simulink library "lib_controls"  (Simulink 7.9)
settings: Solver=ode45  SolverMode=SingleTasking  StartTime=0.0  StopTime=10.0  RelTol=1e-3
undefined symbols (not defined in the file): amb_tmp, cs_charge_deplete_bool, cs_charge_pwr, cs_charge_trq, cs_clt_tmp, cs_decel_fc_off, cs_decel_regen_threshold, cs_dl_assist_trq_threshold, cs_dl_regen_trq_threshold, cs_electric_decel_spd, cs_electric_launch_spd, cs_electric_launch_spd_hi, cs_electric_launch_spd_lo, cs_eng_min_spd, cs_eng_on_soc, cs_fc_init_state, cs_fc_max_pwr_frac, cs_fc_min_pwr_frac, cs_fc_on, cs_fc_pwr_opt, cs_fc_spd_opt, cs_fuzzy_fuel_mode, cs_hi_soc, cs_hi_trq_frac, cs_lo_soc, cs_lo_trq_frac, cs_max_gc_spd, cs_max_pwr, cs_max_pwr_fall_rate, cs_max_pwr_rise_rate, cs_mc_assist_max_frac, cs_mc_assist_min_frac, cs_mc_assist_slope, cs_mc_regen_max_frac, cs_mc_regen_min_frac, cs_mc_regen_slope, cs_mean_eff, cs_mean_eff_bool, cs_min_gc_spd, cs_min_off_time, cs_min_pwr, cs_min_trq_frac, cs_mph_avg_time, cs_off_trq_frac, cs_plot_output, cs_pwr, cs_regen_avg_time, cs_scale_factor, cs_shutoff, cs_soc_range, cs_spd, cs_target_soc, cs_trq_to_soc_factor, cvt_locus_pwr, cvt_locus_spd, cyc_mph, enable_sim_stop_distance, enable_sim_stop_max_spd, enable_sim_stop_speed, enable_sim_stop_time ... (+110)
libraries: lib_controls x124, simulink3 x18, lib_etc x1
(part 13 of 17)

== system lib_controls/<vc> par auto s/a/gearbox control for use w/ AT  in parallel sa/downshift  command1 ==
  prev gear number : Inport
  engine load : Inport  Port=2
  engine speed : Inport  Port=3
  Mux : Mux  Inputs=2
  Relational Operator : RelationalOperator  Operator=>  InputSameDT=on
  load fraction : Subsystem  mask(Gear Selector){spd=gb_dnshift_spd, load=gb_dnshift_load}
      mask prompts: spd "Speeds:"; load "Load Fractions:"
      mask help:
      | This block will perform a linear interplation (extrapolation outside of bounds) to determine the shift point load fraction associated with the current gear number and speed.
      |
      | The Speeds parameter should be defined as an array of vectors containing speeds for each gear number.  The Load Fractions parameter should be defined as a array of vectors containing load fractions indexed by the speeds in the Speeds parameter for each gear number.
      mask Help:
      | Reference the base workspace variables - gb_**shift_spd and gb_**shift_load  where ** is either up for upshift conditions or dn for downshift conditions.
      | 
      | Or define the arrays as follows:
      | 
      | {[spd1 spd2 spd3 spd4]; [spd1 spd2 spd3 spd4]; ...}
      | 
      | {[load1 load2 load3 load4]; [load1 load2 load3 load4]; ...}
      | 
      | where each array contains one row for each gear in the gearbox.  Speeds should be defined in rad/s and loads as a decimal fraction.
  command : Outport  InitialOutput=0
  wires:
  engine speed/1 -> Mux/2
  load fraction/1(Out1) -> Relational Operator/2
  Mux/1 -> load fraction/1(In1)
  engine load/1 -> Relational Operator/1
  prev gear number/1 -> Mux/1
  Relational Operator/1 -> command/1

== system lib_controls/<vc> par auto s/a/gearbox control for use w/ AT  in parallel sa/est. engine trq and spd ==
  prev gear number : Inport
  " prev eta_gb" : Inport  Port=2
  gb_trq_out_r : Inport  Port=3
  gb_spd_out_r : Inport  Port=4
  Block NOTES : Subsystem
      mask Display: disp('Block\nNOTES')
  Constant2 : Constant  Value=[1 1]
  Constant5 : Constant  Value=0
  Demux : Demux  Outputs=2
  K_adv : Subsystem
  Logical Operator : Logic
  Logical Operator1 : Logic  Operator=NOT  Inputs=1
  Memory : Memory
  Mux1 : Mux  Inputs=2
  Mux2 : Mux  Inputs=2
  Relational Operator1 : RelationalOperator  Operator=>  InputSameDT=on
  SR Look-Up Table SR=wout/win : Lookup  InputValues=htc_k_adv  Table=htc_sr  SaturateOnIntegerOverflow=on
  Saturation1 : Saturate  UpperLimit=1  LowerLimit=0.7
  Saturation2 : Saturate  UpperLimit=inf  LowerLimit=0
  Switch : Switch  Threshold=eps  SaturateOnIntegerOverflow=on  InputSameDT=on
  TR Look-Up Table TR=Tout/Tin : Lookup  InputValues=htc_k_adv  Table=htc_tr  SaturateOnIntegerOverflow=on
  TR,SR : Mux  Inputs=2
  gear ratio1 : Lookup  InputValues=[1:length(gb_ratio)]  Table=gb_ratio  SaturateOnIntegerOverflow=on
  ~eng trq and spd : Product  Inputs=*/  SaturateOnIntegerOverflow=on  RndMeth=Zero  InputSameDT=on  OutDataTypeStr=Inherit: Same as first input
  ~gb_spd_in_r : Product  SaturateOnIntegerOverflow=on  RndMeth=Zero  InputSameDT=on  OutDataTypeStr=Inherit: Same as first input
  ~gb_trq_in_r : Product  Inputs=//*  SaturateOnIntegerOverflow=on  RndMeth=Zero  InputSameDT=on  OutDataTypeStr=Inherit: Same as first input
  est eng trq (Nm) : Outport
  est eng spd (rad/s) : Outport  Port=2
  gb_spd_in_est (rad/s)1 : Outport  Port=3
  wires:
  ~gb_spd_in_r/1 -> Mux2/2, gb_spd_in_est (rad/s)1/1, Mux1/2
  ~gb_trq_in_r/1 -> Relational Operator1/1, Mux1/1, Mux2/1
  SR Look-Up Table SR=wout/win/1 -> TR,SR/2
  TR Look-Up Table TR=Tout/Tin/1 -> TR,SR/1
  K_adv/1(K_adv) -> SR Look-Up Table SR=wout/win/1, TR Look-Up Table TR=Tout/Tin/1
  Mux2/1 -> K_adv/1("Req'd output trq and spd (Nm), (rad/s)")
  ~eng trq and spd/1 -> Demux/1
  Mux1/1 -> ~eng trq and spd/1
  [locked_up] -> Memory/1
  Logical Operator/1 -> Switch/2
  Logical Operator1/1 -> Logical Operator/2
  Memory/1 -> Logical Operator1/1
  Demux/1 -> est eng trq (Nm)/1
  prev gear number/1 -> gear ratio1/1
  Relational Operator1/1 -> Logical Operator/1
  Constant5/1 -> Relational Operator1/2
  Saturation2/1 -> est eng spd (rad/s)/1
  Demux/2 -> Saturation2/1
  Saturation1/1 -> ~gb_trq_in_r/2
  " prev eta_gb"/1 -> Saturation1/1
  Switch/1 -> ~eng trq and spd/2
  Constant2/1 -> Switch/3
  TR,SR/1 -> Switch/1
  gear ratio1/1 -> ~gb_spd_in_r/1, ~gb_trq_in_r/1
  gb_spd_out_r/1 -> ~gb_spd_in_r/2
  gb_trq_out_r/1 -> ~gb_trq_in_r/3

== system lib_controls/<vc> par auto s/a/gearbox control for use w/ AT  in parallel sa/est. engine trq and spd assuming lockup ==
  new gear number : Inport
  " prev eta_gb" : Inport  Port=2
  gb_trq_out_r : Inport  Port=3
  gb_spd_in_est : Inport  Port=4
  Block NOTES : Subsystem
      mask Display: disp('Block\nNOTES')
  Memory : Memory  X0=gb_ratio(1)
  Saturation1 : Saturate  UpperLimit=1  LowerLimit=0.7
  Saturation2 : Saturate  UpperLimit=inf  LowerLimit=0
  gear ratio1 : Lookup  InputValues=[1:length(gb_ratio)]  Table=gb_ratio  SaturateOnIntegerOverflow=on
  ~gb_spd_in_r : Product  Inputs=*/*  SaturateOnIntegerOverflow=on  RndMeth=Zero  InputSameDT=on  OutDataTypeStr=Inherit: Same as first input
  ~gb_trq_in_r : Product  Inputs=//*  SaturateOnIntegerOverflow=on  RndMeth=Zero  InputSameDT=on  OutDataTypeStr=Inherit: Same as first input
  est eng trq (Nm) : Outport
  est eng spd (rad/s) : Outport  Port=2
  wires:
  ~gb_spd_in_r/1 -> Saturation2/1
  ~gb_trq_in_r/1 -> est eng trq (Nm)/1
  gb_spd_in_est/1 -> ~gb_spd_in_r/3
  Memory/1 -> ~gb_spd_in_r/2
  Saturation2/1 -> est eng spd (rad/s)/1
  new gear number/1 -> gear ratio1/1
  gb_trq_out_r/1 -> ~gb_trq_in_r/3
  gear ratio1/1 -> Memory/1, ~gb_spd_in_r/1, ~gb_trq_in_r/1
  " prev eta_gb"/1 -> Saturation1/1
  Saturation1/1 -> ~gb_trq_in_r/2

== system lib_controls/<vc> par auto s/a/gearbox control for use w/ AT  in parallel sa/shifting1 ==
  gear number : Inport
  Constant : Constant  Value=gb_shift_delay-1e-6
  Relational Operator : RelationalOperator  Operator=<  InputSameDT=on
  time since last shift : Subsystem
      mask Display: disp('time since\nlast shift')
  out_1 : Outport  InitialOutput=0
  wires:
  Relational Operator/1 -> out_1/1
  gear number/1 -> time since last shift/1(in_1)
  Constant/1 -> Relational Operator/2
  time since last shift/1(out_1) -> Relational Operator/1

== system lib_controls/<vc> par auto s/a/gearbox control for use w/ AT  in parallel sa/upshift  command ==
  prev gear number : Inport
  engine load : Inport  Port=2
  engine speed : Inport  Port=3
  Mux : Mux  Inputs=2
  Relational Operator : RelationalOperator  Operator=<  InputSameDT=on
  load fraction : Subsystem  mask(Gear Selector){spd=gb_upshift_spd, load=gb_upshift_load}
      mask prompts: spd "Speeds:"; load "Load Fractions:"
      mask help:
      | This block will perform a linear interplation (extrapolation outside of bounds) to determine the shift point load fraction associated with the current gear number and speed.
      |
      | The Speeds parameter should be defined as an array of vectors containing speeds for each gear number.  The Load Fractions parameter should be defined as a array of vectors containing load fractions indexed by the speeds in the Speeds parameter for each gear number.
      mask Help:
      | Reference the base workspace variables - gb_**shift_spd and gb_**shift_load  where ** is either up for upshift conditions or dn for downshift conditions.
      | 
      | Or define the arrays as follows:
      | 
      | {[spd1 spd2 spd3 spd4]; [spd1 spd2 spd3 spd4]; ...}
      | 
      | {[load1 load2 load3 load4]; [load1 load2 load3 load4]; ...}
      | 
      | where each array contains one row for each gear in the gearbox.  Speeds should be defined in rad/s and loads as a decimal fraction.
  command : Outport  InitialOutput=0
  wires:
  Relational Operator/1 -> command/1
  engine speed/1 -> Mux/2
  Mux/1 -> load fraction/1(In1)
  prev gear number/1 -> Mux/1
  engine load/1 -> Relational Operator/1
  load fraction/1(Out1) -> Relational Operator/2

== system lib_controls/<vc> par auto s/a/motor controller logic/Block NOTES ==
  note: This block models a motor/controller's logic, modulating the power input requirement as follows:
      | - enforcing the maximum current limit of the motor/controller
      | - shutting the motor off if the average speed over the time step ==0
      | - shutting the motor off if the transmission is shifting.

== system lib_controls/<vc> par auto s/a/motor controller logic/Sign ==
  in_1 : Inport
  Constant : Constant  Value=0
  Relational Operator : RelationalOperator  Operator=>  InputSameDT=on
  Relational Operator1 : RelationalOperator  Operator=<  InputSameDT=on
  Sum : Sum  Inputs=+-  SaturateOnIntegerOverflow=on  InputSameDT=on  OutDataTypeStr=Inherit: Same as first input
  out_1 : Outport  InitialOutput=0
  wires:
  in_1/1 -> Relational Operator/1, Relational Operator1/1
  Constant/1 -> Relational Operator1/2, Relational Operator/2
  Relational Operator1/1 -> Sum/2
  Relational Operator/1 -> Sum/1
  Sum/1 -> out_1/1

== system lib_controls/<vc> par balanced/engine on (balanced parallel hybrid)/Block NOTES1 ==
  note: Engine is on if,
      | 1) engine was on previously and engine is not warm
      | 2) engine was on and is shifting
      | 3) battery power is insufficient
      | 4) (speed is less than electric launch speed OR soc is less than
      | lo soc unless charge depleting) AND
      | soc is less than hi soc AND
      | trq frac is greater than lo trq frac OR soc is less than mean of hi and
      | lo soc unless charge depleting AND
      | (trq is too high AND speed is too high for idle) OR engine is allowed to idle

== system lib_controls/<vc> par balanced/engine on (balanced parallel hybrid)/Subsystem ==
  in_1 : Inport
  Clock : Clock
  Constant1 : Constant  Value=n
  Constant2 : Constant
  Integrator : Integrator
  Memory : Memory  X0=-0.1
  Memory1 : Memory
  Product : Product  Inputs=*/  SaturateOnIntegerOverflow=on  RndMeth=Zero  InputSameDT=on  OutDataTypeStr=Inherit: Same as first input
  Product1 : Product  SaturateOnIntegerOverflow=on  RndMeth=Zero  InputSameDT=on  OutDataTypeStr=Inherit: Same as first input
  Relational Operator : RelationalOperator  Operator=<=  InputSameDT=on
  Sum : Sum  Inputs=+-  SaturateOnIntegerOverflow=on  InputSameDT=on  OutDataTypeStr=Inherit: Same as first input
  Sum1 : Sum  Inputs=|+-  SaturateOnIntegerOverflow=on  InputSameDT=on  OutDataTypeStr=Inherit: Same as first input
  Switch{,1..3} (4 alike) : Switch  Threshold=eps  SaturateOnIntegerOverflow=on  InputSameDT=on
  Variable Transport Delay : VariableTransportDelay  MaximumDelay=n
  out_1 : Outport  InitialOutput=0
  wires:
  Product/1 -> out_1/1
  Sum/1 -> Product/1
  Variable Transport Delay/1 -> Sum/2
  Integrator/1 -> Variable Transport Delay/1, Sum/1
  Relational Operator/1 -> Switch/2
  Constant1/1 -> Product1/2
  Clock/1 -> Sum1/1, Memory/1, Relational Operator/1, Switch/1
  Memory/1 -> Sum1/2
  Sum1/1 -> Product1/1
  Product1/1 -> Relational Operator/2, Switch/3
  Switch/1 -> Variable Transport Delay/2, Switch1/2, Switch1/1
  Constant2/1 -> Switch1/3
  Switch1/1 -> Product/2
  Switch2/1 -> Integrator/1
  Switch3/1 -> Memory1/1
  in_1/1 -> Switch2/3, Switch3/3
  Memory1/1 -> Switch2/1, Switch3/1
  [shifting] -> Switch2/2, Switch3/2

== system lib_controls/<vc> par balanced/engine on (balanced parallel hybrid)/key_on ==
  Clock : Clock
  Fcn1 : Fcn  Expr=rem(u[1],period)
  Look-Up Table : Lookup  InputValues=t  Table=y  SaturateOnIntegerOverflow=on
  out_1 : Outport  InitialOutput=0
  wires:
  Fcn1/1 -> Look-Up Table/1
  Clock/1 -> Fcn1/1
  Look-Up Table/1 -> out_1/1

== system lib_controls/<vc> par balanced/engine on (balanced parallel hybrid)/repeated cycle:  speed required at end of NEXT step ==
  Clock : Clock
  Fcn1 : Fcn  Expr=rem(u[1],period)
  Look-Up Table : Lookup  InputValues=t  Table=y  SaturateOnIntegerOverflow=on
  Memory : Memory  X0=-0.1
  Sum : Sum  Inputs=+-  SaturateOnIntegerOverflow=on  InputSameDT=on  OutDataTypeStr=Inherit: Same as first input
  Sum1 : Sum  SaturateOnIntegerOverflow=on  InputSameDT=on  OutDataTypeStr=Inherit: Same as first input
  out_1 : Outport  InitialOutput=0
  wires:
  Clock/1 -> Sum/1, Memory/1, Fcn1/1
  Memory/1 -> Sum/2
  Sum/1 -> Sum1/2
  Fcn1/1 -> Sum1/1
  Look-Up Table/1 -> out_1/1
  Sum1/1 -> Look-Up Table/1

== system lib_controls/<vc> par balanced/motor controller logic/Block NOTES ==
  note: This block models a motor/controller's logic, modulating the power input requirement as follows:
      | - enforcing the maximum current limit of the motor/controller
      | - shutting the motor off if the average speed over the time step ==0
      | - shutting the motor off if the transmission is shifting.

== system lib_controls/<vc> par balanced/motor controller logic/Sign ==
  in_1 : Inport
  Constant : Constant  Value=0
  Relational Operator : RelationalOperator  Operator=>  InputSameDT=on
  Relational Operator1 : RelationalOperator  Operator=<  InputSameDT=on
  Sum : Sum  Inputs=+-  SaturateOnIntegerOverflow=on  InputSameDT=on  OutDataTypeStr=Inherit: Same as first input
  out_1 : Outport  InitialOutput=0
  wires:
  in_1/1 -> Relational Operator/1, Relational Operator1/1
  Constant/1 -> Relational Operator1/2, Relational Operator/2
  Relational Operator1/1 -> Sum/2
  Relational Operator/1 -> Sum/1
  Sum/1 -> out_1/1

== system lib_controls/<vc> par balanced/parallel clutch control/Block NOTES ==
  note: This clutch control block determines the clutch state given the req'd clutch output torque
      | and speed (labelled as gearbox input torque and speed), and the gear number history.
      |                           conditions                                                                       clutch state
      | gear is being shifted OR (trq <~ 0 AND (engine is                                     1 == disengaged
      | clutched to avoid compression braking OR spd < idle))
      |
      | (trq >~ 0) AND (spd < launch speed) AND clutch                                       2 == slipping
      | was not engaged during previous time step
      |
      | neither of above sets of conditions are met                                          3 == engaged
      |
      | But the clutch is always disengaged when the engine is off or was off within the past 0.5 s.

== system lib_controls/<vc> par balanced/parallel clutch control/gearbox speed estimator ==
  gb_spd_in_r if no gear change : Inport
  Block NOTES : Subsystem
      mask Display: disp('Block\nNOTES')
  Constant : Constant  Value=eps
  Constant1 : Constant  Value=0
  Constant2 : Constant
  Constant3 : Constant  Value=0.11
  Gain : Gain  Gain=0.447  SaturateOnIntegerOverflow=on  OutDataTypeStr=Inherit: Same as input  ParamDataTypeStr=Inherit: Same as input
  Logical : Logic
  Memory : Memory  X0=cyc_mph(1,2)*0.447/wh_radius*fd_ratio*gb_ratio(gb_num_init)
  Memory1 : Memory  X0=1
  Product : Product  Inputs=**/  SaturateOnIntegerOverflow=on  RndMeth=Zero  InputSameDT=on  OutDataTypeStr=Inherit: Same as first input
  Relational : RelationalOperator  Operator=>  InputSameDT=on
  Relational1 : RelationalOperator  Operator=<=  InputSameDT=on
  Sum : Sum  SaturateOnIntegerOverflow=on  InputSameDT=on  OutDataTypeStr=Inherit: Same as first input
  Sum1 : Sum  Inputs=-+  SaturateOnIntegerOverflow=on  InputSameDT=on  OutDataTypeStr=Inherit: Same as first input
  Switch : Switch  Threshold=eps  SaturateOnIntegerOverflow=on  InputSameDT=on
  Switch1 : Switch  Threshold=eps  SaturateOnIntegerOverflow=on  InputSameDT=on
  dt : Subsystem
  Out1 : Outport
  wires:
  dt/1(Out1) -> Relational1/1
  Logical/1 -> Switch1/2
  Memory1/1 -> Logical/1
  Relational1/1 -> Logical/2
  Constant3/1 -> Relational1/2
  [gb_spd_in_a] -> Product/1
  gb_spd_in_r if no gear change/1 -> Switch1/3
  Switch1/1 -> Out1/1
  Switch/1 -> Memory/1
  Relational/1 -> Memory1/1
  Sum1/1 -> Relational/1
  Constant2/1 -> Relational/2
  [mpha] -> Sum1/1, Gain/1
  [cyc_mph_r] -> Sum1/2
  Constant/1 -> Sum/2
  Memory/1 -> Switch1/1
  Constant1/1 -> Switch/3
  [veh_spd_a_rec] -> Switch/2, Sum/1
  Gain/1 -> Product/2
  Sum/1 -> Product/3
  Product/1 -> Switch/1

== system lib_controls/<vc> par balanced/pre-TX parallel gearbox control/Block NOTES ==
  note: This gearbox control block computes the current gear number given the gearbox's
      | req'd output torque and speed and an estimate its efficiency.  Upshifts occur, given a
      | certain engine speed,  when the estimated engine load falls below the upshift curve
      | in engine speed/load space, and downshifts likewise occur when estimated engine
      | load rises above the downshift curve.  Separate upshift and downshift curves are
      | defined for each gear.  An upshift may not be immediately followed by a downshift.
      | If the tires are about to slip, don't upshift unless the engine would be at max. speed.
      | Enforce this rule by setting the load to 1 when the tires are about to slip.

== system lib_controls/<vc> par balanced/pre-TX parallel gearbox control/allow downshift? ==
  prev gearnum : Inport
  Logical Operator : Logic  Operator=NOR
  Memory : Memory  X0=1
  Memory1 : Memory  X0=1
  Relational Operator1 : RelationalOperator  Operator=>  InputSameDT=on
  Relational Operator2 : RelationalOperator  Operator=>  InputSameDT=on
  allow shift : Outport  InitialOutput=0
  wires:
  Relational Operator2/1 -> Logical Operator/2
  Memory1/1 -> Relational Operator2/2
  Memory/1 -> Memory1/1, Relational Operator1/2
  Relational Operator1/1 -> Logical Operator/1
  prev gearnum/1 -> Relational Operator2/1, Memory/1, Relational Operator1/1
  Logical Operator/1 -> allow shift/1

== system lib_controls/<vc> par balanced/pre-TX parallel gearbox control/allow upshift? ==
  prev gearnum : Inport
  gb_trq_out_r : Inport  Port=2
  gb_spd_out_r : Inport  Port=3
  prev Pout/Pin : Inport  Port=4
  Block NOTES1 : Subsystem
      mask Display: disp('Block\nNOTES')
  Constant : Constant
  Constant1 : Constant  Value=max(mc_map_spd)*mc_spd_scale/tc_mc_to_fc_ratio*.95
  Logical Operator1 : Logic  Operator=OR  Inputs=3
  Memory : Memory  X0=1
  Product : Product  SaturateOnIntegerOverflow=on  RndMeth=Zero  InputSameDT=on  OutDataTypeStr=Inherit: Same as first input
  Relational Operator : RelationalOperator  Operator=>  InputSameDT=on
  Relational Operator1 : RelationalOperator  Operator=>  InputSameDT=on
  Saturation : Saturate  UpperLimit=gb_gears_num  LowerLimit=1
  Sum : Sum  SaturateOnIntegerOverflow=on  InputSameDT=on  OutDataTypeStr=Inherit: Same as first input
  est. req'd input pwr (W) : Product  Inputs=**/  SaturateOnIntegerOverflow=on  RndMeth=Zero  InputSameDT=on  OutDataTypeStr=Inherit: Same as first input
  gear ratio : Lookup  InputValues=[1:length(gb_ratio)]  Table=gb_ratio  SaturateOnIntegerOverflow=on
  gear ratio1 : Lookup  InputValues=[1:length(gb_ratio)]  Table=gb_ratio  SaturateOnIntegerOverflow=on
  motor torque capability : Lookup  InputValues=mc_map_spd*mc_spd_scale  Table=mc_max_trq*mc_trq_scale*mc_overtrq_factor+eps  SaturateOnIntegerOverflow=on
  motor (input to gb) pwr capability : Product  SaturateOnIntegerOverflow=on  RndMeth=Zero  InputSameDT=on  OutDataTypeStr=Inherit: Same as first input
  req'd input spd if no gear change : Product  SaturateOnIntegerOverflow=on  RndMeth=Zero  InputSameDT=on  OutDataTypeStr=Inherit: Same as first input
  allow shift : Outport  InitialOutput=0
  wires:
  Memory/1 -> Logical Operator1/2
  [engine_on] -> Memory/1
  Relational Operator/1 -> Logical Operator1/1
  Logical Operator1/1 -> allow shift/1
  prev Pout/Pin/1 -> est. req'd input pwr (W)/3
  gb_trq_out_r/1 -> est. req'd input pwr (W)/2
  est. req'd input pwr (W)/1 -> Relational Operator/2
  motor (input to gb) pwr capability/1 -> Relational Operator/1
  Product/1 -> motor (input to gb) pwr capability/1, motor torque capability/1
  motor torque capability/1 -> motor (input to gb) pwr capability/2
  gear ratio/1 -> Product/1
  Saturation/1 -> gear ratio/1
  Sum/1 -> Saturation/1
  Constant/1 -> Sum/2
  gear ratio1/1 -> req'd input spd if no gear change/1
  prev gearnum/1 -> Sum/1, gear ratio1/1
  gb_spd_out_r/1 -> est. req'd input pwr (W)/1, Product/2, req'd input spd if no gear change/2
  Relational Operator1/1 -> Logical Operator1/3
  Constant1/1 -> Relational Operator1/2
  req'd input spd if no gear change/1 -> Relational Operator1/1

== system lib_controls/<vc> par balanced/pre-TX parallel gearbox control/downshift  command ==
  prev gear number : Inport
  engine load : Inport  Port=2
  engine speed : Inport  Port=3
  Mux : Mux  Inputs=2
  Relational Operator : RelationalOperator  Operator=>  InputSameDT=on
  load fraction : Subsystem  mask(Gear Selector){spd=gb_dnshift_spd, load=gb_dnshift_load}
      mask prompts: spd "Speeds:"; load "Load Fractions:"
      mask help:
      | This block will perform a linear interplation (extrapolation outside of bounds) to determine the shift point load fraction associated with the current gear number and speed.
      |
      | The Speeds parameter should be defined as an array of vectors containing speeds for each gear number.  The Load Fractions parameter should be defined as a array of vectors containing load fractions indexed by the speeds in the Speeds parameter for each gear number.
      mask Help:
      | Reference the base workspace variables - gb_**shift_spd and gb_**shift_load  where ** is either up for upshift conditions or dn for downshift conditions.
      | 
      | Or define the arrays as follows:
      | 
      | {[spd1 spd2 spd3 spd4]; [spd1 spd2 spd3 spd4]; ...}
      | 
      | {[load1 load2 load3 load4]; [load1 load2 load3 load4]; ...}
      | 
      | where each array contains one row for each gear in the gearbox.  Speeds should be defined in rad/s and loads as a decimal fraction.
  command : Outport  InitialOutput=0
  wires:
  load fraction/1(Out1) -> Relational Operator/2
  Mux/1 -> load fraction/1(In1)
  engine load/1 -> Relational Operator/1
  prev gear number/1 -> Mux/1
  engine speed/1 -> Mux/2
  Relational Operator/1 -> command/1

== system lib_controls/<vc> par balanced/pre-TX parallel gearbox control/gearbox speed estimator ==
  gb_spd_in_r if no gear change : Inport
  Block NOTES : Subsystem
      mask Display: disp('Block\nNOTES')
  Constant : Constant  Value=eps
  Constant1 : Constant  Value=0
  Constant2 : Constant  Value=2
  Constant3 : Constant  Value=0.11
  Gain : Gain  Gain=0.447  SaturateOnIntegerOverflow=on  OutDataTypeStr=Inherit: Same as input  ParamDataTypeStr=Inherit: Same as input
  Logical : Logic
  Memory : Memory  X0=cyc_mph(1,2)*0.447/wh_radius*fd_ratio*gb_ratio(gb_num_init)
  Memory1 : Memory  X0=1
  Product : Product  Inputs=**/  SaturateOnIntegerOverflow=on  RndMeth=Zero  InputSameDT=on  OutDataTypeStr=Inherit: Same as first input
  Relational : RelationalOperator  Operator=>  InputSameDT=on
  Relational1 : RelationalOperator  Operator=<=  InputSameDT=on
  Sum : Sum  SaturateOnIntegerOverflow=on  InputSameDT=on  OutDataTypeStr=Inherit: Same as first input
  Sum1 : Sum  Inputs=-+  SaturateOnIntegerOverflow=on  InputSameDT=on  OutDataTypeStr=Inherit: Same as first input
  Switch : Switch  Threshold=eps  SaturateOnIntegerOverflow=on  InputSameDT=on
  Switch1 : Switch  Threshold=eps  SaturateOnIntegerOverflow=on  InputSameDT=on
  dt : Subsystem
  Out1 : Outport
  wires:
  dt/1(Out1) -> Relational1/1
  Logical/1 -> Switch1/2
  Memory1/1 -> Logical/1
  Relational1/1 -> Logical/2
  Constant3/1 -> Relational1/2
  [gb_spd_in_a] -> Product/1
  gb_spd_in_r if no gear change/1 -> Switch1/3
  Switch1/1 -> Out1/1
  Switch/1 -> Memory/1
  Relational/1 -> Memory1/1
  Sum1/1 -> Relational/1
  Constant2/1 -> Relational/2
  [mpha] -> Sum1/1, Gain/1
  [cyc_mph_r] -> Sum1/2
  Constant/1 -> Sum/2
  Memory/1 -> Switch1/1
  Constant1/1 -> Switch/3
  [veh_spd_a_rec] -> Switch/2, Sum/1
  Gain/1 -> Product/2
  Sum/1 -> Product/3
  Product/1 -> Switch/1

== system lib_controls/<vc> par balanced/pre-TX parallel gearbox control/shifting1 ==
  gear number : Inport
  Constant : Constant  Value=gb_shift_delay-1e-6
  Relational Operator : RelationalOperator  Operator=<  InputSameDT=on
  time since last shift : Subsystem
      mask Display: disp('time since\nlast shift')
  out_1 : Outport  InitialOutput=0
  wires:
  Relational Operator/1 -> out_1/1
  gear number/1 -> time since last shift/1(in_1)
  Constant/1 -> Relational Operator/2
  time since last shift/1(out_1) -> Relational Operator/1

== system lib_controls/<vc> par balanced/pre-TX parallel gearbox control/upshift  command ==
  prev gear number : Inport
  engine load : Inport  Port=2
  engine speed : Inport  Port=3
  Mux : Mux  Inputs=2
  Relational Operator : RelationalOperator  Operator=<  InputSameDT=on
  load fraction : Subsystem  mask(Gear Selector){spd=gb_upshift_spd, load=gb_upshift_load}
      mask prompts: spd "Speeds:"; load "Load Fractions:"
      mask help:
      | This block will perform a linear interplation (extrapolation outside of bounds) to determine the shift point load fraction associated with the current gear number and speed.
      |
      | The Speeds parameter should be defined as an array of vectors containing speeds for each gear number.  The Load Fractions parameter should be defined as a array of vectors containing load fractions indexed by the speeds in the Speeds parameter for each gear number.
      mask Help:
      | Reference the base workspace variables - gb_**shift_spd and gb_**shift_load  where ** is either up for upshift conditions or dn for downshift conditions.
      | 
      | Or define the arrays as follows:
      | 
      | {[spd1 spd2 spd3 spd4]; [spd1 spd2 spd3 spd4]; ...}
      | 
      | {[load1 load2 load3 load4]; [load1 load2 load3 load4]; ...}
      | 
      | where each array contains one row for each gear in the gearbox.  Speeds should be defined in rad/s and loads as a decimal fraction.
  command : Outport  InitialOutput=0
  wires:
  load fraction/1(Out1) -> Relational Operator/2
  engine load/1 -> Relational Operator/1
  prev gear number/1 -> Mux/1
  Mux/1 -> load fraction/1(In1)
  engine speed/1 -> Mux/2
  Relational Operator/1 -> command/1

== system lib_controls/<vc> par cvt/cvt control/Block NOTES ==
  note: This CVT control block determines the
      | operating mode of the vehicle
      | and the best gear ratio for that operating mode.
      | For more info on the operating mode selection see
      | block notes in mode selector.
      |
      | The gear ratio is based on the pwr required and an
      | Ideal Operating Line for each mode.  This IOL typically
      | puts the component in its most efficient operating point
      |  for the given power request.

== system lib_controls/<vc> par cvt/cvt control/Mode Selector ==
  SOC : Inport
  trq req : Inport  Port=2
  pwr req : Inport  Port=3
  1=> motor regen 2=> motor only 3=> engine only 4=> engine and motor : Fcn  Expr=u[2]*1+u[1]*u[4]*!u[2]*2+((!u[1]*!u[2]+!u[3]*!u[4])>0)*3+u[1]*u[3]*4
  Block NOTES : Subsystem
      mask Display: disp('Block\nNOTES')
  Constant3 : Constant  Value=-1e-3
  Logical Operator8 : Logic  Operator=OR
  Memory : Memory  X0=cyc_mph(1,2)>0
  Memory1 : Memory  X0=cyc_mph(1,2)>0
  Mux : Mux
  Product : Product  Inputs=/*  SaturateOnIntegerOverflow=on  RndMeth=Zero  InputSameDT=on  OutDataTypeStr=Inherit: Same as first input
  Relational Operator5 : RelationalOperator  Operator=<  InputSameDT=on
  Relational Operator6 : RelationalOperator  Operator=<  InputSameDT=on
  Relational Operator7 : RelationalOperator  Operator=>  InputSameDT=on
  Relational Operator9 : RelationalOperator  Operator=>  InputSameDT=on
  Saturation1 : Saturate  UpperLimit=4  LowerLimit=1
  Saturation2 : Saturate  UpperLimit=2  LowerLimit=1
  Switch4 : Switch  Threshold=eps  SaturateOnIntegerOverflow=on  InputSameDT=on
  cs_fc_max_pwr : Constant  Value=cs_fc_max_pwr_frac
  cs_fc_min_pwr : Constant  Value=cs_fc_min_pwr_frac
  cs_lo_soc : Constant  Value=cs_lo_soc
  fc_max_pwr : Constant  Value=max(fc_map_spd*fc_spd_scale.*fc_max_trq*fc_trq_scale)
  Mode : Outport
  wires:
  Saturation1/1 -> Switch4/1
  1=> motor regen 2=> motor only 3=> engine only 4=> engine and motor/1 -> Saturation2/1, Saturation1/1
  Switch4/1 -> Mode/1
  Saturation2/1 -> Switch4/3
  Product/1 -> Relational Operator7/1, Relational Operator6/1
  Mux/1 -> 1=> motor regen 2=> motor only 3=> engine only 4=> engine and motor/1
  Relational Operator6/1 -> Mux/4
  Relational Operator7/1 -> Mux/3
  Relational Operator9/1 -> Mux/1
  cs_fc_max_pwr/1 -> Relational Operator7/2
  cs_fc_min_pwr/1 -> Relational Operator6/2
  fc_max_pwr/1 -> Product/1
  pwr req/1 -> Product/2
  Logical Operator8/1 -> Switch4/2, Memory/1
  Memory1/1 -> Logical Operator8/1
  [engine_on_cmd] -> Memory1/1
  Memory/1 -> Logical Operator8/2
  Relational Operator5/1 -> Mux/2
  Constant3/1 -> Relational Operator5/2
  trq req/1 -> Relational Operator5/1
  SOC/1 -> Relational Operator9/1
  cs_lo_soc/1 -> Relational Operator9/2

== system lib_controls/<vc> par cvt/cvt control/Speed Interp ==
  Mode : Inport
  pwr req : Inport  Port=2
  Multiport Switch : MultiPortSwitch  Inputs=4  zeroidx=off  SaturateOnIntegerOverflow=on  InputSameDT=on
  Saturation3 : Saturate  UpperLimit=max(ptc_fc_mc_iol_pwr_vec)  LowerLimit=min(ptc_fc_mc_iol_pwr_vec)
  Saturation6 : Saturate  UpperLimit=max(ptc_mc_iol_pwr_vec)  LowerLimit=min(ptc_mc_iol_pwr_vec)
  Saturation7 : Saturate  UpperLimit=max(ptc_fc_iol_pwr_vec)  LowerLimit=min(ptc_fc_iol_pwr_vec)
  Saturation8 : Saturate  UpperLimit=max(ptc_mc_gen_iol_pwr_vec)  LowerLimit=min(ptc_mc_gen_iol_pwr_vec)
  desired engine spd engine and motor : Lookup  InputValues=ptc_fc_mc_iol_pwr_vec  Table=ptc_fc_mc_iol_spd_vec  SaturateOnIntegerOverflow=on
  desired engine spd engine only : Lookup  InputValues=ptc_fc_iol_pwr_vec  Table=ptc_fc_iol_spd_vec  SaturateOnIntegerOverflow=on
  desired motor spd motor only : Lookup  InputValues=ptc_mc_iol_pwr_vec  Table=ptc_mc_iol_spd_vec  SaturateOnIntegerOverflow=on
  desired motor spd motor only regen : Lookup  InputValues=fliplr(ptc_mc_gen_iol_pwr_vec)  Table=fliplr(ptc_mc_gen_iol_spd_vec)  SaturateOnIntegerOverflow=on
  input spd : Outport
  wires:
  desired engine spd engine and motor/1 -> Multiport Switch/5
  desired engine spd engine only/1 -> Multiport Switch/4
  desired motor spd motor only/1 -> Multiport Switch/3
  desired motor spd motor only regen/1 -> Multiport Switch/2
  pwr req/1 -> Saturation8/1, Saturation6/1, Saturation7/1, Saturation3/1
  Mode/1 -> Multiport Switch/1
  Multiport Switch/1 -> input spd/1
  Saturation3/1 -> desired engine spd engine and motor/1
  Saturation7/1 -> desired engine spd engine only/1
  Saturation8/1 -> desired motor spd motor only regen/1
  Saturation6/1 -> desired motor spd motor only/1

== system lib_controls/<vc> par cvt/cvt control/chg pwr req'd (W) ==
  Constant : Constant  Value=cs_charge_pwr*fc_trq_scale
  Goal : Constant  Value=(cs_lo_soc+cs_hi_soc)/2
  Product : Product  SaturateOnIntegerOverflow=on  RndMeth=Zero  InputSameDT=on  OutDataTypeStr=Inherit: Same as first input
  Product1 : Product  Inputs=*/  SaturateOnIntegerOverflow=on  RndMeth=Zero  InputSameDT=on  OutDataTypeStr=Inherit: Same as first input
  Range : Constant  Value=(cs_hi_soc-cs_lo_soc)/2
  Saturation : Saturate  UpperLimit=inf  LowerLimit=-inf
  Sum : Sum  Inputs=-+  SaturateOnIntegerOverflow=on  InputSameDT=on  OutDataTypeStr=Inherit: Same as first input
  add'l pwr req'd (W) : Outport
  wires:
  Saturation/1 -> add'l pwr req'd (W)/1
  Product/1 -> Saturation/1
  Constant/1 -> Product/1
  Product1/1 -> Product/2
  Sum/1 -> Product1/1
  Range/1 -> Product1/2
  Goal/1 -> Sum/2
  [SOC] -> Sum/1

== system lib_controls/<vc> par cvt/cvt control/mod pwr req ==
  In1 : Inport
  Sum : Sum  SaturateOnIntegerOverflow=on  InputSameDT=on  OutDataTypeStr=Inherit: Same as first input
  Out1 : Outport
  wires:
  In1/1 -> Sum/1
  Sum/1 -> Out1/1
  [acc_mech_pwr_est] -> Sum/2

== system lib_controls/<vc> par cvt/engine on (parallel CVT hybrid)/Subsystem ==
  in_1 : Inport
  Clock : Clock
  Constant1 : Constant  Value=n
  Constant2 : Constant
  Integrator : Integrator
  Memory : Memory  X0=-0.1
  Memory1 : Memory
  Product : Product  Inputs=*/  SaturateOnIntegerOverflow=on  RndMeth=Zero  InputSameDT=on  OutDataTypeStr=Inherit: Same as first input
  Product1 : Product  SaturateOnIntegerOverflow=on  RndMeth=Zero  InputSameDT=on  OutDataTypeStr=Inherit: Same as first input
  Relational Operator : RelationalOperator  Operator=<=  InputSameDT=on
  Sum : Sum  Inputs=+-  SaturateOnIntegerOverflow=on  InputSameDT=on  OutDataTypeStr=Inherit: Same as first input
  Sum1 : Sum  Inputs=|+-  SaturateOnIntegerOverflow=on  InputSameDT=on  OutDataTypeStr=Inherit: Same as first input
  Switch{,1..3} (4 alike) : Switch  Threshold=eps  SaturateOnIntegerOverflow=on  InputSameDT=on
  Variable Transport Delay : VariableTransportDelay  MaximumDelay=n
  out_1 : Outport  InitialOutput=0
  wires:
  Product/1 -> out_1/1
  Sum/1 -> Product/1
  Variable Transport Delay/1 -> Sum/2
  Integrator/1 -> Variable Transport Delay/1, Sum/1
  Relational Operator/1 -> Switch/2
  Constant1/1 -> Product1/2
  Clock/1 -> Sum1/1, Memory/1, Relational Operator/1, Switch/1
  Memory/1 -> Sum1/2
  Sum1/1 -> Product1/1
  Product1/1 -> Relational Operator/2, Switch/3
  Switch/1 -> Variable Transport Delay/2, Switch1/2, Switch1/1
  Constant2/1 -> Switch1/3
  Switch1/1 -> Product/2
  Switch2/1 -> Integrator/1
  Switch3/1 -> Memory1/1
  in_1/1 -> Switch2/3, Switch3/3
  Memory1/1 -> Switch2/1, Switch3/1
  [shifting] -> Switch2/2, Switch3/2

== system lib_controls/<vc> par cvt/engine on (parallel CVT hybrid)/key_on ==
  Clock : Clock
  Fcn1 : Fcn  Expr=rem(u[1],period)
  Look-Up Table : Lookup  InputValues=t  Table=y  SaturateOnIntegerOverflow=on
  out_1 : Outport  InitialOutput=0
  wires:
  Fcn1/1 -> Look-Up Table/1
  Clock/1 -> Fcn1/1
  Look-Up Table/1 -> out_1/1

== system lib_controls/<vc> par cvt/engine on (parallel CVT hybrid)/repeated cycle:  speed required at end of NEXT step ==
  Clock : Clock
  Fcn1 : Fcn  Expr=rem(u[1],period)
  Look-Up Table : Lookup  InputValues=t  Table=y  SaturateOnIntegerOverflow=on
  Memory : Memory  X0=-0.1
  Sum : Sum  Inputs=+-  SaturateOnIntegerOverflow=on  InputSameDT=on  OutDataTypeStr=Inherit: Same as first input
  Sum1 : Sum  SaturateOnIntegerOverflow=on  InputSameDT=on  OutDataTypeStr=Inherit: Same as first input
  out_1 : Outport  InitialOutput=0
  wires:
  Sum1/1 -> Look-Up Table/1
  Look-Up Table/1 -> out_1/1
  Fcn1/1 -> Sum1/1
  Sum/1 -> Sum1/2
  Memory/1 -> Sum/2
  Clock/1 -> Fcn1/1, Memory/1, Sum/1

== system lib_controls/<vc> par cvt/motor controller logic/Block NOTES ==
  note: This block models a motor/controller's logic, modulating the power input requirement as follows:
      | - enforcing the maximum current limit of the motor/controller
      | - shutting the motor off if the average speed over the time step ==0
      | - shutting the motor off if the transmission is shifting.

== system lib_controls/<vc> par cvt/motor controller logic/Sign ==
  in_1 : Inport
  Constant : Constant  Value=0
  Relational Operator : RelationalOperator  Operator=>  InputSameDT=on
  Relational Operator1 : RelationalOperator  Operator=<  InputSameDT=on
  Sum : Sum  Inputs=+-  SaturateOnIntegerOverflow=on  InputSameDT=on  OutDataTypeStr=Inherit: Same as first input
  out_1 : Outport  InitialOutput=0
  wires:
  Sum/1 -> out_1/1
  Relational Operator/1 -> Sum/1
  Relational Operator1/1 -> Sum/2
  Constant/1 -> Relational Operator/2, Relational Operator1/2
  in_1/1 -> Relational Operator1/1, Relational Operator/1

== system lib_controls/<vc> par cvt/parallel clutch control/Block NOTES ==
  note: This clutch control block determines the clutch state given the req'd clutch output torque
      | and speed (labelled as gearbox input torque and speed), and the gear number history.
      |                           conditions                                                                       clutch state
      | gear is being shifted OR (trq <~ 0 AND (engine is                                     1 == disengaged
      | clutched to avoid compression braking OR spd < idle))
      |
      | (trq >~ 0) AND (spd < launch speed) AND clutch                                       2 == slipping
      | was not engaged during previous time step
      |
      | neither of above sets of conditions are met                                          3 == engaged
      |
      | But the clutch is always disengaged when the engine is off or was off within the past 0.5 s.

== system lib_controls/<vc> par cvt/parallel clutch control/gearbox speed estimator ==
  gb_spd_in_r if no gear change : Inport
  Block NOTES : Subsystem
      mask Display: disp('Block\nNOTES')
  Constant : Constant  Value=eps
  Constant1 : Constant  Value=0
  Constant2 : Constant
  Constant3 : Constant  Value=0.11
  Gain : Gain  Gain=0.447  SaturateOnIntegerOverflow=on  OutDataTypeStr=Inherit: Same as input  ParamDataTypeStr=Inherit: Same as input
  Logical : Logic
  Memory : Memory  X0=cyc_mph(1,2)*0.447/wh_radius*fd_ratio*gb_ratio(gb_num_init)
  Memory1 : Memory  X0=1
  Product : Product  Inputs=**/  SaturateOnIntegerOverflow=on  RndMeth=Zero  InputSameDT=on  OutDataTypeStr=Inherit: Same as first input
  Relational : RelationalOperator  Operator=>  InputSameDT=on
  Relational1 : RelationalOperator  Operator=<=  InputSameDT=on
  Sum : Sum  SaturateOnIntegerOverflow=on  InputSameDT=on  OutDataTypeStr=Inherit: Same as first input
  Sum1 : Sum  Inputs=-+  SaturateOnIntegerOverflow=on  InputSameDT=on  OutDataTypeStr=Inherit: Same as first input
  Switch : Switch  Threshold=eps  SaturateOnIntegerOverflow=on  InputSameDT=on
  Switch1 : Switch  Threshold=eps  SaturateOnIntegerOverflow=on  InputSameDT=on
  dt : Subsystem
  Out1 : Outport
  wires:
  Product/1 -> Switch/1
  Sum/1 -> Product/3
  Gain/1 -> Product/2
  [veh_spd_a_rec] -> Sum/1, Switch/2
  Constant1/1 -> Switch/3
  Memory/1 -> Switch1/1
  Constant/1 -> Sum/2
  [cyc_mph_r] -> Sum1/2
  [mpha] -> Gain/1, Sum1/1
  Constant2/1 -> Relational/2
  Sum1/1 -> Relational/1
  Relational/1 -> Memory1/1
  Switch/1 -> Memory/1
  Switch1/1 -> Out1/1
  gb_spd_in_r if no gear change/1 -> Switch1/3
  [gb_spd_in_a] -> Product/1
  Constant3/1 -> Relational1/2
  Relational1/1 -> Logical/2
  Memory1/1 -> Logical/1
  Logical/1 -> Switch1/2
  dt/1(Out1) -> Relational1/1

== system lib_controls/<vc> prius/Coordinated  Controller/Block NOTES ==
  note: Hybrid Main Control

== system lib_controls/<vc> prius/Coordinated  Controller/battery charge demand ==
  SOC : Inport
  Memory : Memory  X0=300
  Product2 : Product  SaturateOnIntegerOverflow=on  RndMeth=Zero  InputSameDT=on  OutDataTypeStr=Inherit: Same as first input
  Sum : Sum  Inputs=+-  SaturateOnIntegerOverflow=on  InputSameDT=on  OutDataTypeStr=Inherit: Same as first input
  To Workspace2 : ToWorkspace  VariableName=vc_p_ch_r  SampleTime=-1
  curve fit : Gain  Gain=88  SaturateOnIntegerOverflow=on  OutDataTypeStr=Inherit: Same as input  ParamDataTypeStr=Inherit: Same as input
  gen/mot. eff. : Gain  Gain=1/0.85  SaturateOnIntegerOverflow=on  OutDataTypeStr=Inherit: Same as input  ParamDataTypeStr=Inherit: Same as input
  target soc : Constant  Value=cs_target_soc
  Pch : Outport  InitialOutput=0
  wires:
  Sum/1 -> curve fit/1
  target soc/1 -> Sum/1
  SOC/1 -> Sum/2
  curve fit/1 -> Product2/1  "I"
  gen/mot. eff./1 -> To Workspace2/1, Pch/1
  Product2/1 -> gen/mot. eff./1
  [bus_voltage] -> Memory/1
  Memory/1 -> Product2/2

== system lib_controls/<vc> prius/Coordinated  Controller/max engine efficiency point ==
  pwr requested : Inport
  req ring  speed(rad/s) : Inport  Port=2
  Pch : Inport  Port=3
  Constant : Constant  Value=0
  Constant1 : Constant  Value=0
  Max fc spd (rad/s) : Subsystem
  Min fc spd(rad/s) : Subsystem
  MinMax1 : MinMax  Function=max  Inputs=2  SaturateOnIntegerOverflow=on  InputSameDT=on
  MinMax2 : MinMax  Inputs=2  SaturateOnIntegerOverflow=on  InputSameDT=on
  MinMax3 : MinMax  Inputs=2  SaturateOnIntegerOverflow=on  InputSameDT=on
  Product : Product  Inputs=*/  SaturateOnIntegerOverflow=on  RndMeth=Zero  InputSameDT=on  OutDataTypeStr=Inherit: Same as first input
  Product1 : Product  Inputs=**  SaturateOnIntegerOverflow=on  RndMeth=Zero  InputSameDT=on  OutDataTypeStr=Inherit: Same as first input
  Sum : Sum  SaturateOnIntegerOverflow=on  InputSameDT=on  OutDataTypeStr=Inherit: Same as first input
  Switch1 : Switch  Threshold=eps  SaturateOnIntegerOverflow=on  InputSameDT=on
  Switch2 : Switch  Threshold=eps  SaturateOnIntegerOverflow=on  InputSameDT=on
  Terminator : Terminator
  To Workspace2 : ToWorkspace  VariableName=fc_pwr_out_r  SampleTime=-1
  To Workspace3 : ToWorkspace  VariableName=fc_pwr_out_r2  SampleTime=-1
  at least  idle speed : Subsystem
  cranking? : Subsystem
  fuel on? : Subsystem
  max engine if pwr req>limit : Subsystem
  max_torque lookup : Lookup  InputValues=fc_map_spd*fc_spd_scale  Table=fc_max_trq*fc_trq_scale  SaturateOnIntegerOverflow=on
  need engine on? : Subsystem
  spd opt : Subsystem
  fc_trq_request : Outport  InitialOutput=0
  fc_spd_request1 : Outport  Port=2  InitialOutput=0
  tag scope: engine_on=global
  wires:
  fuel on?/1("fuel on? ") -> Terminator/1
  need engine on?/1(fc on=1) -> [engine_on], Switch2/2, Switch1/2, fuel on?/2(need engine on?1), cranking?/1(need engine on?)
  cranking?/1(cranking?) -> fuel on?/1(cranking?)
  pwr requested/1 -> max engine if pwr req>limit/1(pwr req), Sum/1, need engine on?/1(pwr requested)
  Max fc spd (rad/s)/1(Max fc spd rad/s) -> max engine if pwr req>limit/4(max fc spd), MinMax3/2
  max engine if pwr req>limit/2(spd) -> at least  idle speed/2(spd)
  max engine if pwr req>limit/1(trq) -> at least  idle speed/1(trq)
  at least  idle speed/1(trq1) -> Switch1/1
  at least  idle speed/2(spd1) -> Switch2/1
  Constant1/1 -> Switch2/3
  Constant/1 -> Switch1/3
  Switch2/1 -> Product1/1, fc_spd_request1/1
  Switch1/1 -> Product1/2, fc_trq_request/1
  Product1/1 -> To Workspace3/1
  MinMax2/1 -> max engine if pwr req>limit/2(trq req)
  Sum/1 -> Product/1, To Workspace2/1, spd opt/1(pwr req)
  spd opt/1(spd opt) -> MinMax3/1
  Min fc spd(rad/s)/1(min fc spd rad/s) -> MinMax1/2
  MinMax3/1 -> MinMax1/1
  max_torque lookup/1 -> MinMax2/2
  Product/1 -> MinMax2/1
  MinMax1/1 -> max engine if pwr req>limit/3(spd req), max_torque lookup/1, Product/2
  Pch/1 -> Sum/2
  req ring  speed(rad/s)/1 -> Min fc spd(rad/s)/1(mc spd), Max fc spd (rad/s)/1(mc spd)

== system lib_controls/<vc> prius/prius generator  controller logic/Block NOTES ==
  note: This block models a motor/controller's logic, modulating the power input requirement as follows:
      | - enforcing the maximum current limit of the motor/controller
      | - shutting the motor off if the average speed over the time step ==0

== system lib_controls/<vc> prius/prius generator  controller logic/Sign ==
  in_1 : Inport
  Constant : Constant  Value=0
  Relational Operator : RelationalOperator  Operator=>  InputSameDT=on
  Relational Operator1 : RelationalOperator  Operator=<  InputSameDT=on
  Sum : Sum  Inputs=+-  SaturateOnIntegerOverflow=on  InputSameDT=on  OutDataTypeStr=Inherit: Same as first input
  out_1 : Outport  InitialOutput=0
  wires:
  in_1/1 -> Relational Operator/1, Relational Operator1/1
  Constant/1 -> Relational Operator1/2, Relational Operator/2
  Relational Operator1/1 -> Sum/2
  Relational Operator/1 -> Sum/1
  Sum/1 -> out_1/1

== system lib_controls/<vc> prius/prius motor  controller logic/Block NOTES ==
  note: This block models a motor/controller's logic, modulating the power input requirement as follows:
      | - enforcing the maximum current limit of the motor/controller
      | - shutting the motor off if the average speed over the time step ==0
      | - shutting the motor off if the transmission is shifting.

== system lib_controls/<vc> prius/prius motor  controller logic/Sign ==
  in_1 : Inport
  Constant : Constant  Value=0
  Relational Operator : RelationalOperator  Operator=>  InputSameDT=on
  Relational Operator1 : RelationalOperator  Operator=<  InputSameDT=on
  Sum : Sum  Inputs=+-  SaturateOnIntegerOverflow=on  InputSameDT=on  OutDataTypeStr=Inherit: Same as first input
  out_1 : Outport  InitialOutput=0
  wires:
  in_1/1 -> Relational Operator/1, Relational Operator1/1
  Constant/1 -> Relational Operator1/2, Relational Operator/2
  Relational Operator1/1 -> Sum/2
  Relational Operator/1 -> Sum/1
  Sum/1 -> out_1/1

== system lib_controls/<vc> series/gearbox control for series  HV and EV/Block NOTES ==
  note: This gearbox control block computes the current gear number given the gearbox's
      | req'd output torque and speed and an estimate its efficiency.  Upshifts occur, given a
      | certain engine speed,  when the estimated engine load falls below the upshift curve
      | in engine speed/load space, and downshifts likewise occur when estimated engine
      | load rises above the downshift curve.  Separate upshift and downshift curves are
      | defined for each gear.  An upshift may not be immediately followed by a downshift.
      | If the tires are about to slip, don't upshift unless the engine would be at max. speed.
      | Enforce this rule by setting the load to 1 when the tires are about to slip.

== system lib_controls/<vc> series/gearbox control for series  HV and EV/allow downshift? ==
  prev gearnum : Inport
  Logical Operator : Logic  Operator=NOR
  Memory : Memory  X0=1
  Memory1 : Memory  X0=1
  Relational Operator1 : RelationalOperator  Operator=>  InputSameDT=on
  Relational Operator2 : RelationalOperator  Operator=>  InputSameDT=on
  allow shift : Outport  InitialOutput=0
  wires:
  Logical Operator/1 -> allow shift/1
  prev gearnum/1 -> Relational Operator1/1, Memory/1, Relational Operator2/1
  Relational Operator1/1 -> Logical Operator/1
  Memory/1 -> Relational Operator1/2, Memory1/1
  Memory1/1 -> Relational Operator2/2
  Relational Operator2/1 -> Logical Operator/2

== system lib_controls/<vc> series/gearbox control for series  HV and EV/downshift  command ==
  prev gear number : Inport
  engine load : Inport  Port=2
  engine speed : Inport  Port=3
  Mux : Mux  Inputs=2
  Relational Operator : RelationalOperator  Operator=>  InputSameDT=on
  load fraction : Subsystem  mask(Gear Selector){spd=gb_dnshift_spd, load=gb_dnshift_load}
      mask prompts: spd "Speeds:"; load "Load Fractions:"
      mask help:
      | This block will perform a linear interplation (extrapolation outside of bounds) to determine the shift point load fraction associated with the current gear number and speed.
      |
      | The Speeds parameter should be defined as an array of vectors containing speeds for each gear number.  The Load Fractions parameter should be defined as a array of vectors containing load fractions indexed by the speeds in the Speeds parameter for each gear number.
      mask Help:
      | Reference the base workspace variables - gb_**shift_spd and gb_**shift_load  where ** is either up for upshift conditions or dn for downshift conditions.
      | 
      | Or define the arrays as follows:
      | 
      | {[spd1 spd2 spd3 spd4]; [spd1 spd2 spd3 spd4]; ...}
      | 
      | {[load1 load2 load3 load4]; [load1 load2 load3 load4]; ...}
      | 
      | where each array contains one row for each gear in the gearbox.  Speeds should be defined in rad/s and loads as a decimal fraction.
  command : Outport  InitialOutput=0
  wires:
  load fraction/1(Out1) -> Relational Operator/2
  Mux/1 -> load fraction/1(In1)
  engine load/1 -> Relational Operator/1
  prev gear number/1 -> Mux/1
  engine speed/1 -> Mux/2
  Relational Operator/1 -> command/1

== system lib_controls/<vc> series/gearbox control for series  HV and EV/gearbox speed estimator ==
  gb_spd_in_r if no gear change : Inport
  Block NOTES : Subsystem
      mask Display: disp('Block\nNOTES')
  Constant : Constant  Value=eps
  Constant1 : Constant  Value=0
  Constant2 : Constant
  Constant3 : Constant  Value=0.11
  Gain : Gain  Gain=0.447  SaturateOnIntegerOverflow=on  OutDataTypeStr=Inherit: Same as input  ParamDataTypeStr=Inherit: Same as input
  Logical : Logic
  Memory : Memory  X0=cyc_mph(1,2)*0.447/wh_radius*fd_ratio*gb_ratio(gb_num_init)
  Memory1 : Memory  X0=1
  Product : Product  Inputs=**/  SaturateOnIntegerOverflow=on  RndMeth=Zero  InputSameDT=on  OutDataTypeStr=Inherit: Same as first input
  Relational : RelationalOperator  Operator=>  InputSameDT=on
  Relational1 : RelationalOperator  Operator=<=  InputSameDT=on
  Sum : Sum  SaturateOnIntegerOverflow=on  InputSameDT=on  OutDataTypeStr=Inherit: Same as first input
  Sum1 : Sum  Inputs=-+  SaturateOnIntegerOverflow=on  InputSameDT=on  OutDataTypeStr=Inherit: Same as first input
  Switch : Switch  Threshold=eps  SaturateOnIntegerOverflow=on  InputSameDT=on
  Switch1 : Switch  Threshold=eps  SaturateOnIntegerOverflow=on  InputSameDT=on
  dt : Subsystem
  Out1 : Outport
  wires:
  Product/1 -> Switch/1
  Sum/1 -> Product/3
  Gain/1 -> Product/2
  [veh_spd_a_rec] -> Sum/1, Switch/2
  Constant1/1 -> Switch/3
  Memory/1 -> Switch1/1
  Constant/1 -> Sum/2
  [cyc_mph_r] -> Sum1/2
  [mpha] -> Gain/1, Sum1/1
  Constant2/1 -> Relational/2
  Sum1/1 -> Relational/1
  Relational/1 -> Memory1/1
  Switch/1 -> Memory/1
  Switch1/1 -> Out1/1
  gb_spd_in_r if no gear change/1 -> Switch1/3
  [gb_spd_in_a] -> Product/1
  dt/1(Out1) -> Relational1/1
  Memory1/1 -> Logical/1
  Logical/1 -> Switch1/2
  Relational1/1 -> Logical/2
  Constant3/1 -> Relational1/2
